simulink model "helikopter04"  (Simulink 7.5)
settings: Solver=ode1  StartTime=0.0  StopTime=inf  FixedStep=0.001  RelTol=1e-3
values from neighbouring files (symbols this model uses):
  K_ed = 10    [init02.m]    (also in init04.m = 5.5; init05.m)
  K_ei = 2.3    [init02.m]    (also in init04.m = 2.2;2.0; init05.m)
  K_ep = 7    [init02.m]    (also in init04.m = 5; init05.m)
  K_pd = w_c/K_1    (= 13.1840341488)    [init02.m]    (also in init04.m = 5.78737814632; init05.m = 13.8589538532)
  K_pp = (sqrt(2)*w_c^2)/K_1    [init02.m]    (also in init04.m; init05.m)
  KalibElevasjon = .105    (= 0.105)    [init02.m]    (also in init04.m; init05.m)
  KalibPitch = .0879    (= 0.0879)    [init02.m]    (also in init04.m; init05.m)
  KalibVandring = -.0879    (= -0.0879)    [init02.m]    (also in init04.m = -0.088; init05.m = -0.18)
  V_b_eq = .6    (= 0.6)    [init02.m]    (also in init04.m = 0.691; init05.m = 0.707)
  V_f_eq = .635    (= 0.635)    [init02.m]    (also in init04.m = 0.595; init05.m = 0.595)
undefined symbols (not defined in the file or in its folder): HIL
libraries: quarc_library x3
settings Model: Creator=Administrator  LastModifiedBy=jesmanim  SimulationMode=external  ExtModeTrigDuration=10000
settings SolverCC: PositivePriorityOrder=on
settings OptimizationCC: InitFltsAndDblsToZero=on
settings DebuggingCC: StrictBusMsg=Warning
settings RTWCC: SystemTargetFile=quarc_windows.tlc  TemplateMakefile=quarc_default_tmf  Description=QuaRC Win32 Target  ProcessScript=quarc_windows_make_rtw_hook
settings STFCustomTargetCC: TargetPreCompLibLocation=C:\PROGRA~2\QUARC\lib\2010a\windows\release  GeneratePreprocessorConditionals=Disable all  SystemTargetFile=quarc_windows.tlc
settings GRTTargetCC: TargetPreCompLibLocation=C:\PROGRA~2\QUARC\lib\2010a\windows\release  ParMdlRefBuildCompliant=off  CompOptLevelCompliant=off  MatFileLogging=off  ExtMode=on  ExtModeMexFile=quarc_comm

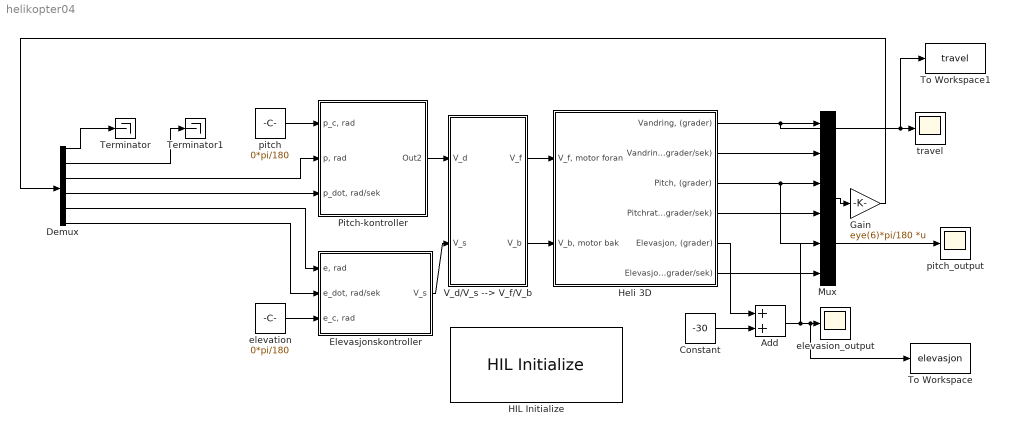
== system helikopter04 ==
  Add : Sum  OutDataType=sfix(16)  OutScaling=2^-10
  Constant : Constant  Value=-30  OutDataType=sfix(16)  OutScaling=2^0
  Demux : Demux  Outputs=6
  Elevasjonskontroller : Subsystem
  Gain : Gain  Gain=eye(6)*pi/180  Multiplication=Matrix(K*u)  ParameterDataType=sfix(16)  ParameterScaling=2^0  OutDataType=sfix(16)  OutScaling=2^0
  HIL Initialize : quarc_library/Data Acquisition/Generic/Configuration/HIL Initialize  object_name=HIL-1  board_type=sensoray_model_626  board_number=0  exclusive=off  active=on  hardware_clocks=[0 1 2 3 4 5]  clock_modes=2  set_clock_params_at_start=on  set_clock_params_at_switch_in=on  analog_input_channels=[0:15]  analog_input_maximums=10  analog_input_minimums=-10  set_analog_input_params_at_start=on  set_analog_input_params_at_switch_in=off  analog_output_channels=[0:3]  analog_output_maximums=10  analog_output_minimums=-10  initial_analog_outputs=[0]  final_analog_outputs=[0]  watchdog_analog_outputs=[]  set_analog_output_params_at_start=off  set_analog_output_params_at_switch_in=off  set_analog_outputs_at_start=on  set_analog_outputs_at_switch_in=off  set_analog_outputs_at_terminate=on  set_analog_outputs_at_switch_out=off  set_analog_outputs_on_watchdog=off  digital_input_channels=[]  digital_output_channels=[]  digital_output_configuration=[]  initial_digital_outputs=[1]  final_digital_outputs=[1]  watchdog_digital_outputs=[]  set_digital_output_params_at_start=off  set_digital_output_params_at_switch_in=off  set_digital_outputs_at_start=on  set_digital_outputs_at_switch_in=off  set_digital_outputs_at_terminate=on  set_digital_outputs_at_switch_out=off  set_digital_outputs_on_watchdog=off  encoder_channels=[]  quadrature=[4]  encoder_filter_frequency=[]  initial_encoder_counts=[0]  set_encoder_params_at_start=on  set_encoder_params_at_switch_in=off  set_encoder_counts_at_start=on  set_encoder_counts_at_switch_in=off  pwm_channels=[]  pwm_modes=[]  pwm_frequency=[]  pwm_configuration=[]  pwm_alignment=[]  pwm_polarity=[]  pwm_leading_deadband=[]  pwm_trailing_deadband=[]  initial_pwm_outputs=[]  final_pwm_outputs=[]  watchdog_pwm_outputs=[]  set_pwm_params_at_start=off  set_pwm_params_at_switch_in=off  set_pwm_outputs_at_start=off  set_pwm_outputs_at_switch_in=off  set_pwm_outputs_at_terminate=off  set_pwm_outputs_at_switch_out=off  set_pwm_outputs_on_watchdog=off  other_output_channels=[]  initial_other_outputs=[]  final_other_outputs=[]  watchdog_other_outputs=[]  set_other_outputs_at_start=off  set_other_outputs_at_switch_in=off  set_other_outputs_at_terminate=off  set_other_outputs_at_switch_out=off  set_other_outputs_on_watchdog=off
  Heli 3D : Subsystem
  Mux : Mux  Inputs=6
  Pitch-kontroller : Subsystem
  Terminator : Terminator
  Terminator1 : Terminator
  To Workspace : ToWorkspace  VariableName=elevasjon  SampleTime=-1  SaveFormat=Structure With Time
  To Workspace1 : ToWorkspace  VariableName=travel  SampleTime=-1  SaveFormat=Structure With Time
  V_d/V_s --> V_f/V_b : Subsystem
  elevasion_output : Scope
      settings: TimeRange=10  YMin=9.875  YMax=10.125
  elevation : Constant  Value=0*pi/180  OutDataType=sfix(16)  OutScaling=2^0
  pitch : Constant  Value=0*pi/180  OutDataType=sfix(16)  OutScaling=2^0
  pitch_output : Scope
      settings: YMin=29.05  YMax=29.65  SaveName=ScopeData3
  travel : Scope
      settings: YMin=5931.5  YMax=5940  SaveName=ScopeData2
  wires:
  Pitch-kontroller/1(Out2) -> V_d/V_s --> V_f/V_b/1(V_d)
  Elevasjonskontroller/1(V_s) -> V_d/V_s --> V_f/V_b/2(V_s)
  Heli 3D/1("Vandring, (grader)") -> Mux/1, travel/1, To Workspace1/1
  Heli 3D/4("Pitchrate, (grader/sek)") -> Mux/4
  Heli 3D/5("Elevasjon, (grader)") -> Add/1
  Heli 3D/6(Elevasjonsrate (grader/sek)) -> Mux/6
  Mux/1 -> Gain/1
  Demux/1 -> Terminator/1
  Demux/2 -> Terminator1/1
  Gain/1 -> Demux/1
  pitch/1 -> Pitch-kontroller/1("p_c, rad")
  Demux/3 -> Pitch-kontroller/2("p, rad")
  Demux/4 -> Pitch-kontroller/3("p_dot, rad/sek")
  Demux/5 -> Elevasjonskontroller/1("e, rad")
  Demux/6 -> Elevasjonskontroller/2("e_dot, rad/sek")
  elevation/1 -> Elevasjonskontroller/3("e_c, rad")
  Constant/1 -> Add/2
  Add/1 -> Mux/5, elevasion_output/1, To Workspace/1
  Heli 3D/3("Pitch, (grader)") -> Mux/3, pitch_output/1
  Heli 3D/2("Vandringsrate, (grader/sek)") -> Mux/2
  V_d/V_s --> V_f/V_b/1(V_f) -> Heli 3D/1("V_f, motor foran")
  V_d/V_s --> V_f/V_b/2(V_b) -> Heli 3D/2("V_b, motor bak")

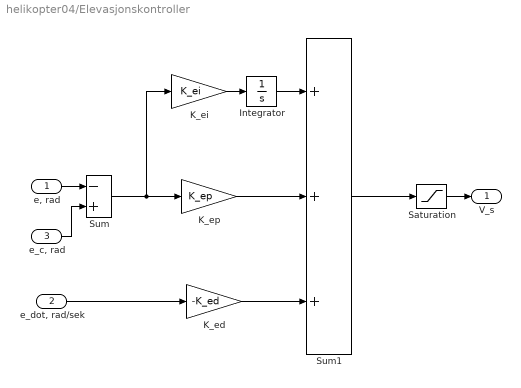
== system helikopter04/Elevasjonskontroller ==
  "e, rad" : Inport
  "e_dot, rad/sek" : Inport  Port=2
  "e_c, rad" : Inport  Port=3
  Integrator : Integrator  LimitOutput=on
  K_ed : Gain  Gain=-K_ed  SaturateOnIntegerOverflow=on  OutDataTypeStr=Inherit: Same as input  ParamDataTypeStr=Inherit: Same as input
  K_ei : Gain  Gain=K_ei  SaturateOnIntegerOverflow=on  OutDataTypeStr=Inherit: Same as input  ParamDataTypeStr=Inherit: Same as input
  K_ep : Gain  Gain=K_ep  SaturateOnIntegerOverflow=on  OutDataTypeStr=Inherit: Same as input  ParamDataTypeStr=Inherit: Same as input
  Saturation : Saturate  UpperLimit=10  LowerLimit=-10
  Sum : Sum  Inputs=-+  SaturateOnIntegerOverflow=on  InputSameDT=on  OutDataTypeStr=Inherit: Same as first input
  Sum1 : Sum  Inputs=+++  SaturateOnIntegerOverflow=on  InputSameDT=on  OutDataTypeStr=Inherit: Same as first input
  V_s : Outport  InitialOutput=0
  wires:
  Sum/1 -> K_ei/1, K_ep/1
  "e, rad"/1 -> Sum/1
  "e_c, rad"/1 -> Sum/2
  "e_dot, rad/sek"/1 -> K_ed/1
  Saturation/1 -> V_s/1
  Sum1/1 -> Saturation/1
  K_ep/1 -> Sum1/2
  K_ed/1 -> Sum1/3
  Integrator/1 -> Sum1/1
  K_ei/1 -> Integrator/1

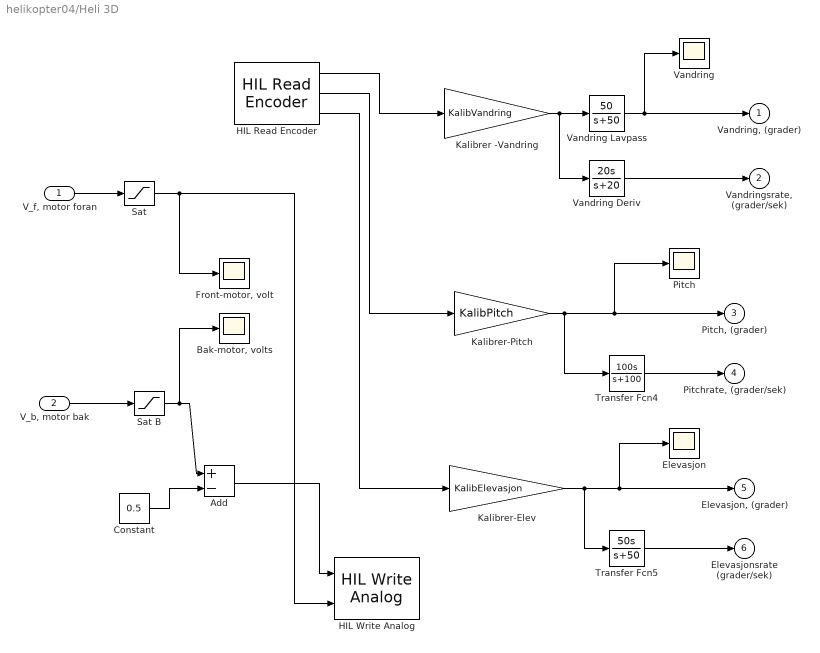
== system helikopter04/Heli 3D ==
  "V_f, motor foran" : Inport
  "V_b, motor bak" : Inport  Port=2
  Add : Sum  Inputs=+-  OutDataType=fixdt(1, 16)  OutScaling=2^-10
  "Bak-motor, volts" : Scope
      settings: TickLabels=on  TimeRange=1.234000  YMin=-1.560000  YMax=1.560000  DataFormat=Array
  Constant : Constant  Value=0.5  OutDataType=sfix(16)  OutScaling=2^0
  Elevasjon : Scope
      settings: TickLabels=on  TimeRange=1.234000  YMin=-1.56  YMax=1.56  DataFormat=Array
  "Front-motor, volt" : Scope
      settings: TickLabels=on  TimeRange=1.234000  YMin=-1.560000  YMax=1.560000  DataFormat=Array
  HIL Read Encoder : quarc_library/Data Acquisition/Generic/Immediate I//O/HIL Read Encoder  object_name=HIL-1  channels=[0,1,2]  sample_time=qc_get_step_size  active=on  vector_output=off  data_type_mode=Inherit via back propagation  data_type=double
  HIL Write Analog : quarc_library/Data Acquisition/Generic/Immediate I//O/HIL Write Analog  object_name=HIL-1  channels=[1,0]  sample_time=-1  active=off  vector_input=off
  Kalibrer -Vandring : Gain  Gain=KalibVandring  SaturateOnIntegerOverflow=on  OutDataTypeStr=Inherit: Same as input  ParamDataTypeStr=Inherit: Same as input
  Kalibrer-Elev : Gain  Gain=KalibElevasjon  SaturateOnIntegerOverflow=on  OutDataTypeStr=Inherit: Same as input  ParamDataTypeStr=Inherit: Same as input
  Kalibrer-Pitch : Gain  Gain=KalibPitch  SaturateOnIntegerOverflow=on  OutDataTypeStr=Inherit: Same as input  ParamDataTypeStr=Inherit: Same as input
  Pitch : Scope
      settings: TickLabels=on  TimeRange=1.000000  YMin=-1  YMax=1  DataFormat=Array
  Sat : Saturate  UpperLimit=5  LowerLimit=-5
  Sat B : Saturate  UpperLimit=5  LowerLimit=-5
  Transfer Fcn4 : TransferFcn  Numerator=[100 0]  Denominator=[1 100]
  Transfer Fcn5 : TransferFcn  Numerator=[50 0]  Denominator=[1 50]
  Vandring : Scope
      settings: TickLabels=on  TimeRange=1.000000  YMin=1  YMax=2.4  DataFormat=Array
  Vandring Deriv : TransferFcn  Numerator=[20 0]  Denominator=[1 20]
  Vandring Lavpass : TransferFcn  Numerator=[50]  Denominator=[1 50]
  "Vandring, (grader)" : Outport  InitialOutput=0
  "Vandringsrate, (grader/sek)" : Outport  Port=2  InitialOutput=0
  "Pitch, (grader)" : Outport  Port=3  InitialOutput=0
  "Pitchrate, (grader/sek)" : Outport  Port=4  InitialOutput=0
  "Elevasjon, (grader)" : Outport  Port=5  InitialOutput=0
  Elevasjonsrate (grader/sek) : Outport  Port=6  InitialOutput=0
  wires:
  Vandring Deriv/1 -> "Vandringsrate, (grader/sek)"/1
  Vandring Lavpass/1 -> Vandring/1, "Vandring, (grader)"/1
  Kalibrer -Vandring/1 -> Vandring Deriv/1, Vandring Lavpass/1
  Kalibrer-Pitch/1 -> Pitch/1, "Pitch, (grader)"/1, Transfer Fcn4/1
  Transfer Fcn4/1 -> "Pitchrate, (grader/sek)"/1
  Kalibrer-Elev/1 -> Transfer Fcn5/1, Elevasjon/1, "Elevasjon, (grader)"/1
  Transfer Fcn5/1 -> Elevasjonsrate (grader/sek)/1
  Sat/1 -> "Front-motor, volt"/1, HIL Write Analog/2
  Sat B/1 -> "Bak-motor, volts"/1, Add/1
  "V_f, motor foran"/1 -> Sat/1
  "V_b, motor bak"/1 -> Sat B/1
  HIL Read Encoder/1 -> Kalibrer -Vandring/1
  HIL Read Encoder/2 -> Kalibrer-Pitch/1
  HIL Read Encoder/3 -> Kalibrer-Elev/1
  Add/1 -> HIL Write Analog/1
  Constant/1 -> Add/2

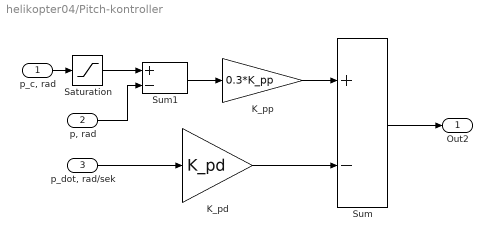
== system helikopter04/Pitch-kontroller ==
  "p_c, rad" : Inport
  "p, rad" : Inport  Port=2
  "p_dot, rad/sek" : Inport  Port=3
  K_pd : Gain  Gain=K_pd  SaturateOnIntegerOverflow=on  OutDataTypeStr=Inherit: Same as input  ParamDataTypeStr=Inherit: Same as input
  K_pp : Gain  Gain=0.3*K_pp  SaturateOnIntegerOverflow=on  OutDataTypeStr=Inherit: Same as input  ParamDataTypeStr=Inherit: Same as input
  Saturation : Saturate  UpperLimit=50*pi/180  LowerLimit=-50*pi/180
  Sum : Sum  Inputs=+-  SaturateOnIntegerOverflow=on  InputSameDT=on  OutDataTypeStr=Inherit: Same as first input
  Sum1 : Sum  Inputs=+-  SaturateOnIntegerOverflow=on  InputSameDT=on  OutDataTypeStr=Inherit: Same as first input
  Out2 : Outport  InitialOutput=0
  wires:
  Saturation/1 -> Sum1/1
  "p_c, rad"/1 -> Saturation/1
  Sum1/1 -> K_pp/1
  Sum/1 -> Out2/1
  K_pp/1 -> Sum/1
  K_pd/1 -> Sum/2
  "p_dot, rad/sek"/1 -> K_pd/1
  "p, rad"/1 -> Sum1/2

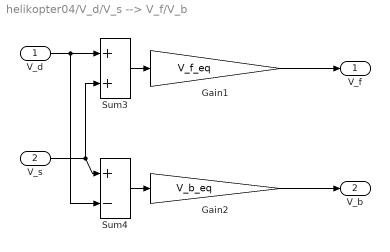
== system helikopter04/V_d/V_s --> V_f/V_b ==
  V_d : Inport
  V_s : Inport  Port=2
  Gain1 : Gain  Gain=V_f_eq  SaturateOnIntegerOverflow=on  OutDataTypeStr=Inherit: Same as input  ParamDataTypeStr=Inherit: Same as input
  Gain2 : Gain  Gain=V_b_eq  SaturateOnIntegerOverflow=on  OutDataTypeStr=Inherit: Same as input  ParamDataTypeStr=Inherit: Same as input
  Sum3 : Sum  SaturateOnIntegerOverflow=on  InputSameDT=on  OutDataTypeStr=Inherit: Same as first input
  Sum4 : Sum  Inputs=+-  SaturateOnIntegerOverflow=on  InputSameDT=on  OutDataTypeStr=Inherit: Same as first input
  V_f : Outport  InitialOutput=0
  V_b : Outport  Port=2  InitialOutput=0
  wires:
  Gain2/1 -> V_b/1
  Gain1/1 -> V_f/1
  V_d/1 -> Sum4/2, Sum3/1
  Sum4/1 -> Gain2/1
  Sum3/1 -> Gain1/1
  V_s/1 -> Sum3/2, Sum4/1
